simulink model "SIGAS_RT_System"  (R2026a)
settings: Solver=ode23t  StopTime=20  MaxStep=0.01  RelTol=1e-4
settings Model: Creator=josue  LastModifiedBy=josue

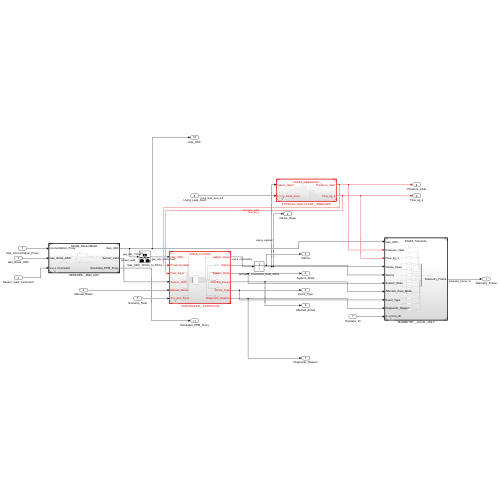
[thumbnail: Simulink's stored preview of the top-level diagram]
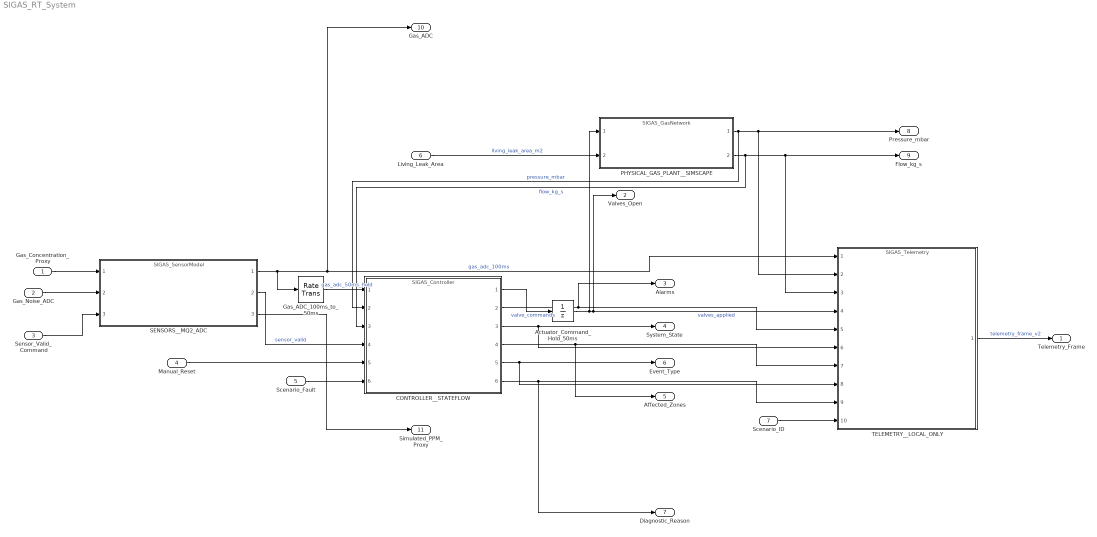
== system SIGAS_RT_System ==
  Gas_Concentration_Proxy : Inport  PortDimensions=3
  Gas_Noise_ADC : Inport  Port=2  PortDimensions=3
  Sensor_Valid_Command : Inport  Port=3  PortDimensions=3
  Manual_Reset : Inport  Port=4  PortDimensions=1
  Scenario_Fault : Inport  Port=5  PortDimensions=1
  Living_Leak_Area : Inport  Port=6  PortDimensions=1
  Scenario_ID : Inport  Port=7  PortDimensions=1
  Actuator_Command_Hold_50ms : UnitDelay  InitialCondition=false(4,1)  SampleTime=0.05
  CONTROLLER__STATEFLOW : ModelReference  ModelNameDialog=SIGAS_Controller  SimulationMode=Normal  ModelReferenceVersion=1.2
  Gas_ADC_100ms_to_50ms : RateTransition  InitialCondition=zeros(3,1)  OutPortSampleTime=0.05
  PHYSICAL_GAS_PLANT__SIMSCAPE : ModelReference  ModelNameDialog=SIGAS_GasNetwork  SimulationMode=Normal  ModelReferenceVersion=1.12
  SENSORS__MQ2_ADC : ModelReference  ModelNameDialog=SIGAS_SensorModel  SimulationMode=Normal  ModelReferenceVersion=1.1
  TELEMETRY__LOCAL_ONLY : ModelReference  ModelNameDialog=SIGAS_Telemetry  SimulationMode=Normal  ModelReferenceVersion=1.3
  Telemetry_Frame : Outport
  Valves_Open : Outport  Port=2
  Alarms : Outport  Port=3
  System_State : Outport  Port=4
  Affected_Zones : Outport  Port=5
  Event_Type : Outport  Port=6
  Diagnostic_Reason : Outport  Port=7
  Pressure_mbar : Outport  Port=8
  Flow_kg_s : Outport  Port=9
  Gas_ADC : Outport  Port=10
  Simulated_PPM_Proxy : Outport  Port=11
  wires:
  SENSORS__MQ2_ADC/3 -> Simulated_PPM_Proxy/1
  Sensor_Valid_Command/1 -> SENSORS__MQ2_ADC/3
  Gas_Noise_ADC/1 -> SENSORS__MQ2_ADC/2
  Gas_Concentration_Proxy/1 -> SENSORS__MQ2_ADC/1
  Gas_ADC_100ms_to_50ms/1 -> CONTROLLER__STATEFLOW/1  "gas_adc_50ms_hold"
  SENSORS__MQ2_ADC/1 -> TELEMETRY__LOCAL_ONLY/1, Gas_ADC/1, Gas_ADC_100ms_to_50ms/1  "gas_adc_100ms"
  PHYSICAL_GAS_PLANT__SIMSCAPE/1 -> Pressure_mbar/1, TELEMETRY__LOCAL_ONLY/2, CONTROLLER__STATEFLOW/2  "pressure_mbar"
  PHYSICAL_GAS_PLANT__SIMSCAPE/2 -> Flow_kg_s/1, TELEMETRY__LOCAL_ONLY/3, CONTROLLER__STATEFLOW/3  "flow_kg_s"
  SENSORS__MQ2_ADC/2 -> CONTROLLER__STATEFLOW/4  "sensor_valid"
  Manual_Reset/1 -> CONTROLLER__STATEFLOW/5
  Scenario_Fault/1 -> CONTROLLER__STATEFLOW/6
  Living_Leak_Area/1 -> PHYSICAL_GAS_PLANT__SIMSCAPE/2  "living_leak_area_m2"
  CONTROLLER__STATEFLOW/2 -> Alarms/1, TELEMETRY__LOCAL_ONLY/5
  CONTROLLER__STATEFLOW/3 -> System_State/1, TELEMETRY__LOCAL_ONLY/6
  CONTROLLER__STATEFLOW/4 -> Affected_Zones/1, TELEMETRY__LOCAL_ONLY/7
  CONTROLLER__STATEFLOW/5 -> Event_Type/1, TELEMETRY__LOCAL_ONLY/8
  CONTROLLER__STATEFLOW/6 -> Diagnostic_Reason/1, TELEMETRY__LOCAL_ONLY/9
  Scenario_ID/1 -> TELEMETRY__LOCAL_ONLY/10
  TELEMETRY__LOCAL_ONLY/1 -> Telemetry_Frame/1  "telemetry_frame_v2"
  Actuator_Command_Hold_50ms/1 -> Valves_Open/1, TELEMETRY__LOCAL_ONLY/4, PHYSICAL_GAS_PLANT__SIMSCAPE/1  "valves_applied"
  CONTROLLER__STATEFLOW/1 -> Actuator_Command_Hold_50ms/1  "valve_commands"
